simulink model "Supersonic_CoTurnHold_Autopilot"  (R2020a)
settings: Solver=VariableStepAuto  StartTime=0.0  StopTime=10.0  RelTol=1e-3
undefined symbols (not defined in the file or in its folder): A, B, C, D
settings Model: Creator=AHSAN  LastModifiedBy=AHSAN

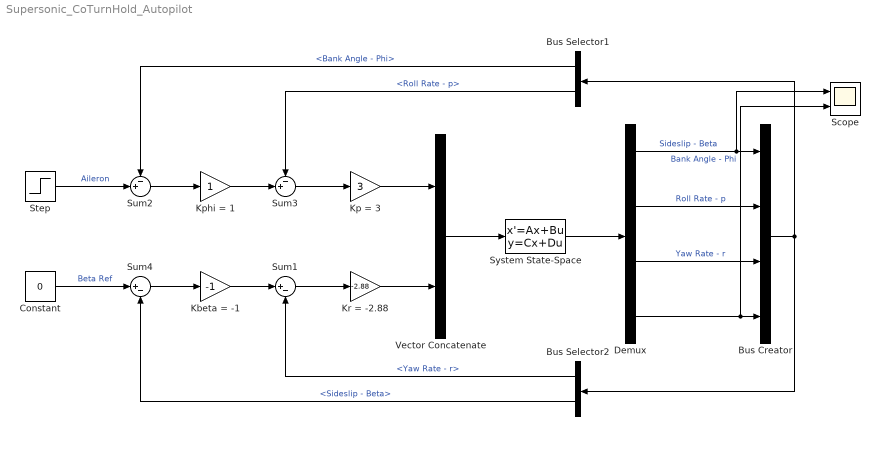
== system Supersonic_CoTurnHold_Autopilot ==
  Bus Creator : BusCreator  Inputs=4
  Bus Selector1 : BusSelector  OutputSignals=Bank Angle - Phi,Roll Rate - p
  Bus Selector2 : BusSelector  OutputSignals=Yaw Rate - r,Sideslip - Beta
  Constant : Constant  Value=0
  Demux : Demux
  Kbeta = -1 : Gain  Gain=-1
  Kp = 3 : Gain  Gain=3
  Kphi = 1 : Gain
  Kr = -2.88 : Gain  Gain=-2.88
  Scope : Scope  NumInputPorts=2
  Step : Step  Time=0  SampleTime=0
  Sum1 : Sum  Inputs=|+-
  Sum2 : Sum  Inputs=-+|
  Sum3 : Sum  Inputs=-+|
  Sum4 : Sum  Inputs=|+-
  System State-Space : StateSpace  A=A  B=B  C=C  D=D  InitialCondition=0
  Vector Concatenate : Concatenate
  wires:
  Sum1/1 -> Kr = -2.88/1
  Kr = -2.88/1 -> Vector Concatenate/2
  Demux/4 -> Bus Creator/4, Scope/2  "Bank Angle - Phi"
  Demux/2 -> Bus Creator/2  "Roll Rate - p"
  Bus Selector2/1 -> Sum1/2  "<Yaw Rate - r>"
  Demux/3 -> Bus Creator/3  "Yaw Rate - r"
  Demux/1 -> Bus Creator/1, Scope/1  "Sideslip - Beta"
  System State-Space/1 -> Demux/1
  Sum3/1 -> Kp = 3/1
  Vector Concatenate/1 -> System State-Space/1
  Bus Selector1/2 -> Sum3/1  "<Roll Rate - p>"
  Kp = 3/1 -> Vector Concatenate/1
  Bus Creator/1 -> Bus Selector2/1, Bus Selector1/1
  Constant/1 -> Sum4/1  "Beta Ref"
  Step/1 -> Sum2/2  "Aileron"
  Sum2/1 -> Kphi = 1/1
  Kphi = 1/1 -> Sum3/2
  Kbeta = -1/1 -> Sum1/1
  Bus Selector2/2 -> Sum4/2  "<Sideslip - Beta>"
  Bus Selector1/1 -> Sum2/1  "<Bank Angle - Phi>"
  Sum4/1 -> Kbeta = -1/1
